simulink model "Fig134"  (R2014a)
settings: Solver=FixedStepDiscrete  StartTime=0.0  StopTime=.05  FixedStep=1.25e-6  RelTol=1e-3
undefined symbols (not defined in the file): fdesignblkfcn, gcbh
libraries: commchan3 x1, commanapbnd3 x1
(part 2 of 2)

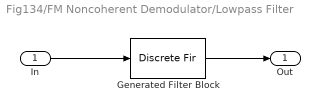
== system Fig134/FM Noncoherent Demodulator/Lowpass Filter ==
  In : Inport
  Generated Filter Block : DiscreteFir  Tag=BlockMethodSubSystem  Coefficients=[0.00049012927714864448 -0.00015443095771300157 -0.0001340205860285048 -0.00011821130629516578 -0.00010528394801493984 -9.5610857531854866e-05 -8.7711751957089885e-05 -8.2172421464364966e-05 -7.7663069831323075e-05 -7.492237786083252e-05 -7.2707485478572037e-05 -7.1877053134816347e-05 -7.1222715068964995e-05 -7.1713886448599145e-05 -7.2121420096729291e-05 -7.3555320270110884e-05 -7.4654418463584158e-05 -7.6910278836686725e-05 -7.8118882854744348e-05 -8.1426117637690824e-05 -8.302526802290175e-05 -8.5506459607171824e-05 -8.8614228036876914e-05 -9.1672995985480287e-05 -9.421302832341718e-05 -9.7174262920201237e-05 -0.00010015794886187028 -0.0001037106630221872 -0.00010696056008402659 -0.00011050479201382473 -0.000113623514562572 -0.00011716252506145501 -0.00012041194327254803 -0.00012422134382381587 -0.00012769933332297458 -0.0001317335762798578 -0.0001352202721898526 -0.00013933170358972459 -0.00014282118317872166 -0.00014673271425472416 -0.00015057688107679673 -0.00015449465890402761 -0.00015824494431637887 -0.00016250730491762196 -0.00016647795602637129 -0.00017070220951055019 -0.00017459559102350492 -0.00017890433271372963 -0.00018290907410701548 -0.00018724327303779514 -0.00019117194882140861 -0.00019546855964004472 -0.00019943711940356018 -0.00020386834662661495 -0.00020793422463190379 -0.0002124272161801537 -0.00021651286716756359 -0.0002209127618490188 -0.00022510338330809099 -0.00022947181208712793 -0.00023361894523832674 -0.00023811389858447254 -0.00024218490478180855 -0.00024653994954621997 -0.00025058660467655521 -0.0002549640903987648 -0.00025895622236455718 -0.00026327782221803012 -0.00026728102005834378 -0.00027164793495889006 -0.0002756295991378982 -0.00027990818453179673 -0.00028378473258394856 -0.00028799378713804301 -0.00029184866023942464 -0.00029596911137944303 -0.00029977866843786252 -0.00030376845258678337 -0.0003074455797230546 -0.00031141424693732945 -0.00031495050192031047 -0.00031878076409761033 -0.0003222265431833046 -0.00032590984967000703 -0.00032917620729762642 -0.00033275521437395225 -0.00033596105556663269 -0.00033943537819739871 -0.00034248741185551686 -0.00034581222557105524 -0.00034873185373386048 -0.00035189640470656972 -0.00035464306620406163 -0.00035760472744498692 -0.00036020740621936731 -0.00036300755260332463 -0.0003654132000187092 -0.00036804337667992816 -0.00037019524575224541 -0.00037261598013631713 -0.00037461116912995506 -0.00037681835433889997 -0.00037858060328140882 -0.00038057540539026597 -0.00038209936590760131 -0.00038382418693905641 -0.00038510421166130918 -0.00038660855796005683 -0.00038765104754411213 -0.00038888130433813997 -0.00038967264264422097 -0.00039066379023277063 -0.00039123179892920726 -0.0003919663373614587 -0.00039224240043748168 -0.0003927225334531512 -0.00039270030131454542 -0.00039289621749095808 -0.00039260114249779798 -0.00039248337835603075 -0.00039190708921161275 -0.00039153477127130433 -0.00039066591757215747 -0.00038997185232796669 -0.00038879976064814002 -0.00038780252346226331 -0.00038632083800982744 -0.00038501885651735963 -0.00038325480685337353 -0.0003816472513267773 -0.00037955664851561385 -0.00037762385069254977 -0.00037521327356771622 -0.0003729920948351734 -0.00037024860822746546 -0.00036769409558514831 -0.00036463737514709976 -0.00036174846969355196 -0.00035838238518674499 -0.0003551843701295052 -0.00035148408066864852 -0.00034796440027385343 -0.00034397008701952155 -0.00034013881015281563 -0.0003358215715661214 -0.00033167923800479619 -0.00032706468205396947 -0.00032260942580120415 -0.0003176760074556629 -0.00031291162694469578 -0.00030765677133229606 -0.00030258289960299927 -0.00029701322700692546 -0.00029165279066537583 -0.00028582005230379568 -0.00028015983982287133 -0.00027403540618319342 -0.00026808765834903568 -0.00026167370143870982 -0.00025545613624363615 -0.0002487810426081741 -0.00024228401132720632 -0.00023534114865199639 -0.00022859940177639174 -0.00022141173304136846 -0.00021441509845077398 -0.00020698263051382109 ...(+32685 chars)]  InputProcessing=Columns as channels (frame based)
  Out : Outport
  wires:
  In/1 -> Generated Filter Block/1
  Generated Filter Block/1 -> Out/1
